simulink model "uloha2_4_ABS_subsystem_mask"  (R2020b)
settings: Solver=VariableStepAuto  StartTime=0.0  StopTime=10  RelTol=1e-3  EnableMultiTasking=on
undefined symbols (not defined in the file or in its folder): g, J, m, mi, r, skluz, v0
settings Model: Creator=Jirkovsk  LastModifiedBy=jirkovsky
settings DataIOCC: LimitDataPoints=on  SaveFormat=Array  ReturnWorkspaceOutputs=off
settings OptimizationCC: ExpressionDepthLimit=2147483647  LifeSpan=inf
settings DebuggingCC: UnderspecifiedInitializationDetection=Classic  MergeDetectMultiDrivingBlocksExec=none  SolverPrmCheckMsg=warning  StateNameClashWarn=warning  SFUnexpectedBacktrackingDiag=warning  SFNoUnconditionalDefaultTransitionDiag=warning  SFExecutionAtInitializationDiag=none  ArithmeticOperatorsInVariantConditions=warning
settings HardwareCC: ProdBitPerPointer=32  ProdBitPerSizeT=32  ProdBitPerPtrDiffT=32  ProdLargestAtomicFloat=None  ProdIntDivRoundTo=Undefined  ProdEndianess=Unspecified  ProdWordSize=32  ProdHWDeviceType=32-bit Generic
settings ModelReferenceCC: PropagateSignalLabelsOutOfModel=off
settings SFSimCC: SimUseLocalCustomCode=off  CustomCodeUndefinedFunction=UseInterfaceOnly
settings RTWCC: RTWUseLocalCustomCode=off
settings CodeAppCC: StateflowObjectComments=on
settings GRTTargetCC: TargetLangStandard=C89/C90 (ANSI)
settings ConfigComp: CovMetricSettings=dw  CovSaveCumulativeToWorkspaceVar=on  CovSaveSingleToWorkspaceVar=on  CovExternalEMLEnable=off

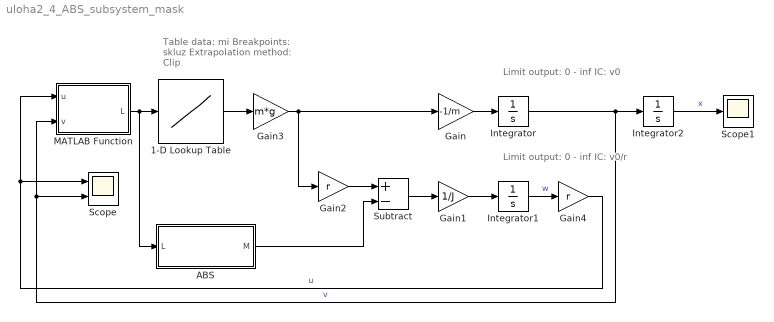
== system uloha2_4_ABS_subsystem_mask ==
  note: Table data: mi
      | Breakpoints: skluz
      | Extrapolation method: Clip
  note: Limit output: 0 - inf
      | IC: v0/r
  note: Limit output: 0 - inf
      | IC: v0
  1-D Lookup Table : Lookup_n-D  NumberOfTableDimensions=1  BreakpointsForDimension1=skluz  Table=mi  ExtrapMethod=Clip  RndMeth=Simplest  InputSameDT=on
  ABS : Subsystem  mask(System ABS){wL=0.19}
      mask prompts: wL "Pozadovany skluz"
      mask help:
      | System Anti-lock Breaking System (ABS) umoznuje brzdeni vozidla bez zablokovani kol. Zadanym parametrem je pozadovany skluz pneumatiky, ktery odpovida vysokemu koeficientu treni.
      |
      |                   u
      |       L = 1 - ----
      |                   v
      |
      | kde L je skluz, u je obvodova rychlost kola a v je rychlost vozidla.
  Gain : Gain  Gain=-1/m
  Gain1 : Gain  Gain=1/J
  Gain2 : Gain  Gain=r
  Gain3 : Gain  Gain=m*g
  Gain4 : Gain  Gain=r
  Integrator : Integrator  InitialCondition=v0  LimitOutput=on  LowerSaturationLimit=0
  Integrator1 : Integrator  InitialCondition=v0/r  LimitOutput=on  LowerSaturationLimit=0
  Integrator2 : Integrator
  MATLAB Function : MATLAB Function  TreatAsAtomicUnit=on
  Scope : Scope  NumInputPorts=2
  Scope1 : Scope
  Subtract : Sum  Inputs=+-
  wires:
  Gain3/1 -> Gain/1, Gain2/1
  Gain/1 -> Integrator/1
  Gain1/1 -> Integrator1/1
  Subtract/1 -> Gain1/1
  Gain2/1 -> Subtract/1
  1-D Lookup Table/1 -> Gain3/1
  MATLAB Function/1(L) -> ABS/1(L), 1-D Lookup Table/1
  Integrator/1 -> MATLAB Function/2(v), Scope/2, Integrator2/1  "v"
  Integrator1/1 -> Gain4/1  "w"
  ABS/1(M) -> Subtract/2
  Integrator2/1 -> Scope1/1  "x"
  Gain4/1 -> MATLAB Function/1(u), Scope/1  "u"

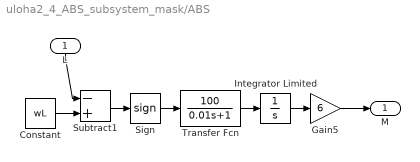
== system uloha2_4_ABS_subsystem_mask/ABS ==
  L : Inport
  Constant : Constant  Value=wL
  Gain5 : Gain  Gain=6
  Integrator Limited : Integrator  LimitOutput=on  UpperSaturationLimit=200  LowerSaturationLimit=0
  Sign : Signum
  Subtract1 : Sum  Inputs=-+
  Transfer Fcn : TransferFcn  Numerator=[100]  Denominator=[0.01 1]
  M : Outport
  wires:
  L/1 -> Subtract1/1
  Constant/1 -> Subtract1/2
  Subtract1/1 -> Sign/1
  Sign/1 -> Transfer Fcn/1
  Transfer Fcn/1 -> Integrator Limited/1
  Integrator Limited/1 -> Gain5/1
  Gain5/1 -> M/1

== matlab function uloha2_4_ABS_subsystem_mask/MATLAB Function ==
  data: u input; L output; v input
function L = fcn(u,v)

L = 1 - u/v;
